simulink model "P_4_3_b_FIFO_LIFO"  (R2020b)
settings: Solver=VariableStepAuto  StartTime=0.0  StopTime=100  RelTol=1e-3
undefined symbols (not defined in the file or in its folder): m, n
settings Model: Creator=csoka  LastModifiedBy=csoka

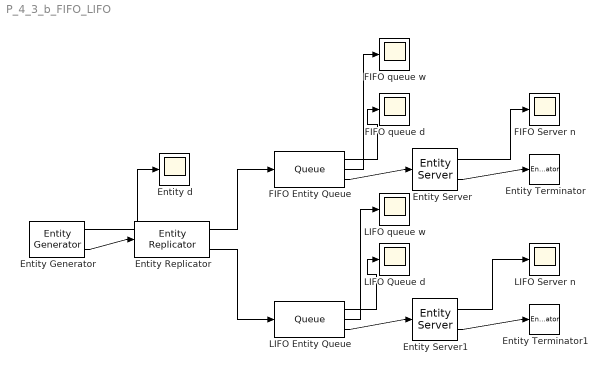
== system P_4_3_b_FIFO_LIFO ==
  Entity Generator : EntityGenerator  OutputPortMessageModes=n,m  TimeSource=MATLAB action  IntergenerationTimeAction=|  NumberEntitiesDeparted=on  EntityType=Structured  EntityTypeName=Entity
      | dt = rand(1,1);
      | persistent rngInit;
      | if isempty(rngInit)
      |     seed = 12345;
      |     rng(seed);
      |     rngInit = true;
      | end
      | 
      | % Pattern: Exponential distribution
      | mu = 1;
      | dt = -mu * log(1 - rand());
      settings: OutputPortMap=o0,o3
  Entity Replicator : EntityReplicator  InputPortMessageModes=m  OutputPortMessageModes=m,m
  Entity Server : EntityServer  InputPortMessageModes=m  OutputPortMessageModes=n,m  Capacity=1  NumberEntitiesInBlock=on
      settings: OutputPortMap=o1,o9
  Entity Server1 : EntityServer  InputPortMessageModes=m  OutputPortMessageModes=n,m  Capacity=1  NumberEntitiesInBlock=on
      settings: OutputPortMap=o1,o9
  Entity Terminator : EntityTerminator  InputPortMessageModes=m
  Entity Terminator1 : EntityTerminator  InputPortMessageModes=m
  Entity d : Scope
  FIFO Entity Queue : Queue  InputPortMessageModes=m  OutputPortMessageModes=n,n,m  NumberEntitiesDeparted=on  AverageWait=on
      settings: OutputPortMap=o0,o2,o5
  FIFO Server n : Scope
  FIFO queue d : Scope
  FIFO queue w : Scope
  LIFO Entity Queue : Queue  InputPortMessageModes=m  OutputPortMessageModes=n,n,m  QueueType=LIFO  NumberEntitiesDeparted=on  AverageWait=on
      settings: OutputPortMap=o0,o2,o5
  LIFO Queue d : Scope
  LIFO Server n : Scope
  LIFO queue w : Scope
  wires:
  LIFO Entity Queue/3 -> Entity Server1/1
  Entity Server1/2 -> Entity Terminator1/1
  Entity Server/2 -> Entity Terminator/1
  FIFO Entity Queue/3 -> Entity Server/1
  Entity Replicator/1 -> FIFO Entity Queue/1
  Entity Replicator/2 -> LIFO Entity Queue/1
  Entity Generator/2 -> Entity Replicator/1
  Entity Server/1 -> FIFO Server n/1
  FIFO Entity Queue/1 -> FIFO queue d/1
  Entity Server1/1 -> LIFO Server n/1
  LIFO Entity Queue/1 -> LIFO Queue d/1
  Entity Generator/1 -> Entity d/1
  FIFO Entity Queue/2 -> FIFO queue w/1
  LIFO Entity Queue/2 -> LIFO queue w/1
